simulink model "two_mass_model"  (R2021b)
settings: Solver=FixedStepAuto  StartTime=0.0  StopTime=0.25  FixedStep=Tq  RelTol=1e-3
values from neighbouring files (symbols this model uses):
  c0 = X(1,1)    [calc_PR.m]    (also in compare_PRs.m = pr_params(1))
  J1 = J1_v(i)    [calc_params_sensivity.m]    (also in compare_PRs.m = J1_nom*Ttest(1,i); compare_steps.m = J1_nom*Ttest(1,vector_num); neuro_net_testing.m = J1_nom*Y(1); test_PR.m = J1_nom*Ttest(1,vector_num))
  noise_level = 0    [compare_PRs.m]    (also in neuro_net_testing.m)
  pref_gain = 10*(C*c0/Ksp + r0)    [calc_params_sensivity.m]    (also in compare_PRs.m; compare_steps.m; neuro_net_testing.m; test_PR.m)
  r0 = X(3,1)    [calc_PR.m]    (also in compare_PRs.m = pr_params(3))
  r1 = X(2,1)    [calc_PR.m]    (also in compare_PRs.m = pr_params(2))
undefined symbols (not defined in the file or in its folder): C, dec_factor, Ksp, Ra, Ta, Tq, Uy
libraries: simulink x1
settings Model: Creator=Ilya  LastModifiedBy=Ilya
settings SolverCC: AlgebraicLoopSolver=TrustRegion
settings DataIOCC: LimitDataPoints=on  SaveFormat=Array  SignalLoggingSaveFormat=ModelDataLogs  ReturnWorkspaceOutputs=off
settings OptimizationCC: BlockReduction=off  BooleanDataType=off  LifeSpan=inf
settings DebuggingCC: SaveWithParameterizedLinksMsg=none  UnderspecifiedInitializationDetection=Classic  MergeDetectMultiDrivingBlocksExec=none  SignalResolutionControl=TryResolveAllWithWarning  MultiTaskDSMMsg=warning  MultiTaskCondExecSysMsg=none  SFUnexpectedBacktrackingDiag=warning  SFNoUnconditionalDefaultTransitionDiag=warning  SFExecutionAtInitializationDiag=none  SFMachineParentedDataDiag=warning  ArithmeticOperatorsInVariantConditions=warning
settings HardwareCC: ProdBitPerPointer=32  ProdBitPerSizeT=32  ProdBitPerPtrDiffT=32  ProdLargestAtomicFloat=None  ProdIntDivRoundTo=Undefined  ProdEndianess=Unspecified  ProdWordSize=32  ProdHWDeviceType=32-bit Generic  TargetUnknown=on
settings ModelReferenceCC: PropagateSignalLabelsOutOfModel=off
settings SFSimCC: SimUseLocalCustomCode=off  CustomCodeUndefinedFunction=UseInterfaceOnly
settings RTWCC: RTWUseLocalCustomCode=off
settings CodeAppCC: StateflowObjectComments=on
settings GRTTargetCC: TargetLangStandard=C89/C90 (ANSI)
settings ConfigComp: CovMetricSettings=dw  CovSaveCumulativeToWorkspaceVar=on  CovSaveSingleToWorkspaceVar=on  CovExternalEMLEnable=off

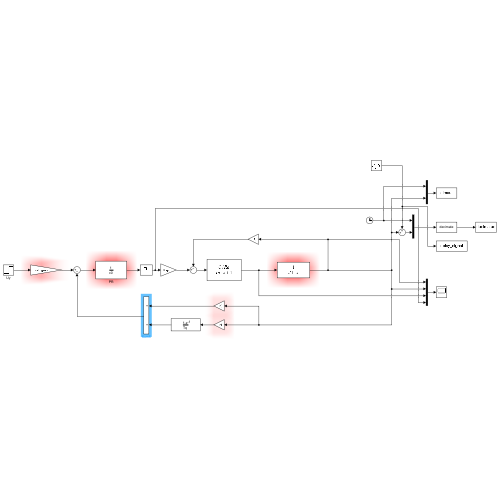
[thumbnail: Simulink's stored preview of the top-level diagram]
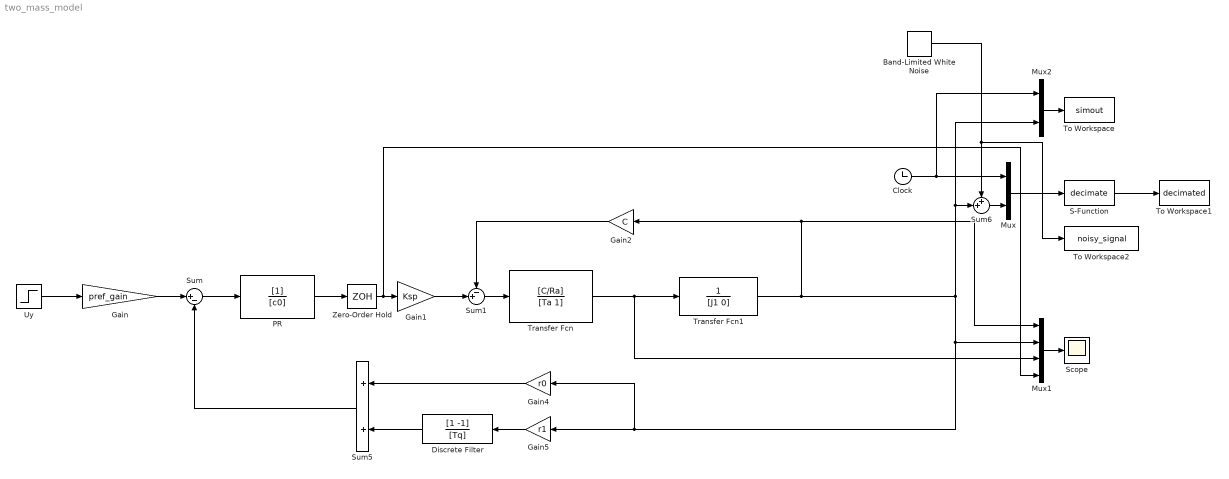
== system two_mass_model ==
  Band-Limited White Noise : simulink/Sources/Band-Limited White Noise  Cov=[noise_level]  Ts=Tq  seed=[23341]
  Clock : Clock
  Discrete Filter : DiscreteFilter  Numerator=[1 -1]  Denominator=[Tq]  SampleTime=Tq
  Gain : Gain  Gain=pref_gain
  Gain1 : Gain  Gain=Ksp
  Gain2 : Gain  Gain=C
  Gain4 : Gain  Gain=r0  SampleTime=Tq
  Gain5 : Gain  Gain=r1  SampleTime=Tq
  Mux : Mux  Inputs=2
  Mux1 : Mux
  Mux2 : Mux  Inputs=2
  PR : DiscreteFilter  Denominator=[c0]  SampleTime=Tq
  S-Function : S-Function  FunctionName=decimate  Parameters=Tq,dec_factor,Uy  SFunctionDeploymentMode=off  EnableBusSupport=off
  Scope : Scope
  Sum : Sum  Inputs=|+-
  Sum1 : Sum  Inputs=-+|
  Sum5 : Sum  SampleTime=Tq
  Sum6 : Sum  Inputs=++|
  To Workspace : ToWorkspace  VariableName=simout  SampleTime=Tq
  To Workspace1 : ToWorkspace  VariableName=decimated  SampleTime=Tq
      settings: Decimation=dec_factor
  To Workspace2 : ToWorkspace  VariableName=noisy_signal  SampleTime=Tq
  Transfer Fcn : TransferFcn  Numerator=[C/Ra]  Denominator=[Ta 1]
  Transfer Fcn1 : TransferFcn  Denominator=[J1 0]
  Uy : Step  Time=0  After=Uy  SampleTime=0
  Zero-Order Hold : ZeroOrderHold  SampleTime=Tq
  wires:
  Uy/1 -> Gain/1
  Gain/1 -> Sum/1
  Sum/1 -> PR/1
  PR/1 -> Zero-Order Hold/1
  Zero-Order Hold/1 -> Mux1/4, Gain1/1
  Gain1/1 -> Sum1/2
  Sum1/1 -> Transfer Fcn/1
  Transfer Fcn/1 -> Transfer Fcn1/1, Mux1/3
  Gain2/1 -> Sum1/1
  Transfer Fcn1/1 -> Gain2/1, Mux1/1, Gain5/1, Gain4/1, Mux1/2, Mux2/2, Sum6/2
  Gain4/1 -> Sum5/1
  Gain5/1 -> Discrete Filter/1
  Discrete Filter/1 -> Sum5/2
  Sum5/1 -> Sum/2
  Clock/1 -> Mux2/1, Mux/1
  Mux/1 -> S-Function/1
  S-Function/1 -> To Workspace1/1
  Mux1/1 -> Scope/1
  Sum6/1 -> Mux/2
  Band-Limited White Noise/1 -> To Workspace2/1, Sum6/1
  Mux2/1 -> To Workspace/1
